simulink model "DynamicVibrationAbsorber"  (R2019b)
settings: Solver=VariableStepAuto  StartTime=0.0  StopTime=10  MaxStep=0.001  RelTol=1e-3
model workspace (MAT data in the model file):
  K12 = Simulink.Parameter
  K12.Value = 15
  K12.DataType = 'auto'
  K12.Dimensions = [1 1]
  M2 = Simulink.Parameter
  M2.Value = 25
  M2.DataType = 'auto'
  M2.Dimensions = [1 1]
settings Model: OrderedModelArguments=off  Creator=ip  LastModifiedBy=ip

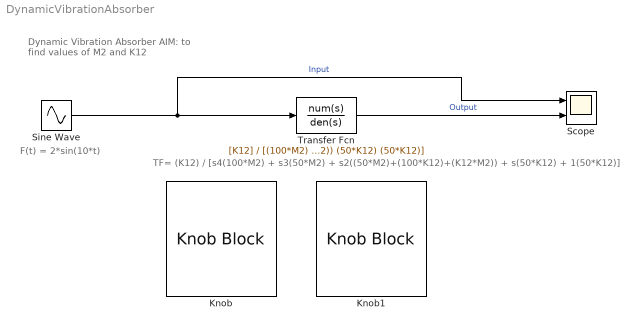
== system DynamicVibrationAbsorber ==
  note: Dynamic Vibration Absorber
      | AIM: to find values of M2 and K12
  note: TF= (K12) / [s4(100*M2) + s3(50*M2) + s2((50*M2)+(100*K12)+(K12*M2)) + s(50*K12) + 1(50*K12)]
  note: F(t) = 2*sin(10*t)
  Knob : KnobBlock
  Knob1 : KnobBlock
  Scope : Scope  NumInputPorts=2
  Sine Wave : Sin  Amplitude=2  Frequency=10  SampleTime=0
  Transfer Fcn : TransferFcn  Numerator=[K12]  Denominator=[(100*M2) (50*M2) ((50*M2)+(100*K12)+(K12*M2)) (50*K12) (50*K12)]
  wires:
  Sine Wave/1 -> Scope/1, Transfer Fcn/1  "Input"
  Transfer Fcn/1 -> Scope/2  "Output"
